simulink model "12_FOC_jieou_fanzhuan_2019b"  (R2019b)
settings: Solver=ode45  StartTime=0.0  StopTime=1  MaxStep=1e-4  RelTol=1e-3  EnableMultiTasking=on
libraries: powerlib x9, simulink x4
settings Model: Creator=uu  LastModifiedBy=李瑾年
settings DataIOCC: LimitDataPoints=on  ReturnWorkspaceOutputs=off
settings OptimizationCC: LifeSpan=inf
settings DebuggingCC: AllowSymbolicDim=off  SFUnexpectedBacktrackingDiag=warning  SFNoUnconditionalDefaultTransitionDiag=warning  ArithmeticOperatorsInVariantConditions=warning
settings ModelReferenceCC: PropagateSignalLabelsOutOfModel=off
settings SFSimCC: SimUseLocalCustomCode=off  CustomCodeUndefinedFunction=UseInterfaceOnly
settings RTWCC: RTWUseLocalCustomCode=off
settings CodeAppCC: StateflowObjectComments=on
settings GRTTargetCC: TargetLangStandard=C89/C90 (ANSI)
settings ConfigComp: CovMetricSettings=dw  CovHtmlReporting=on  CovSaveCumulativeToWorkspaceVar=on  CovSaveSingleToWorkspaceVar=on  CovExternalEMLEnable=off
settings SimscapeCC: SimscapeNormalizeSystem=off

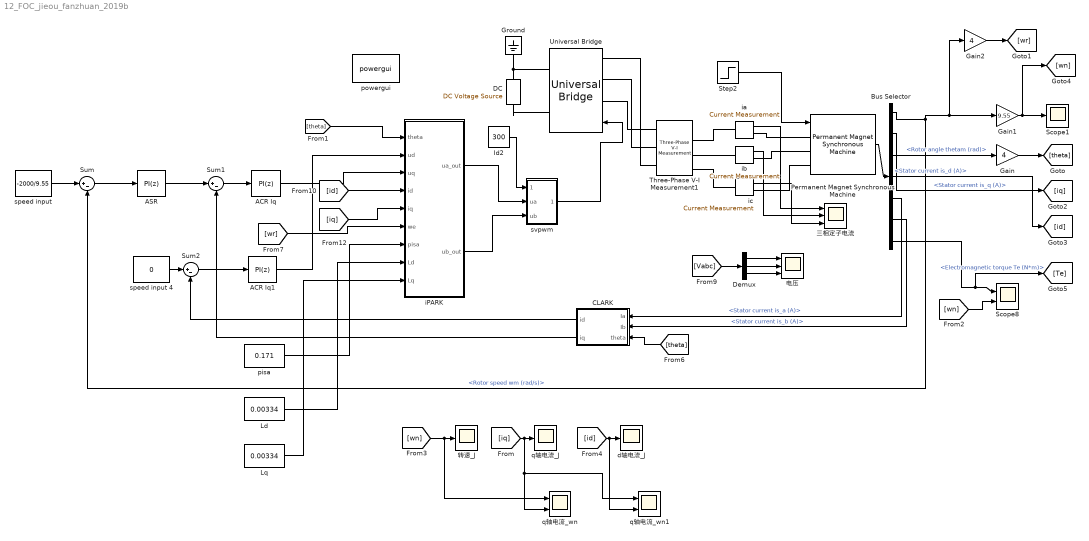
== system 12_FOC_jieou_fanzhuan_2019b ==
  ACR Iq : simulink/Continuous/PID Controller  Controller=PI  Form=Parallel  TimeDomain=Discrete-time  SampleTime=0.0002  IntegratorMethod=Forward Euler  FilterMethod=Forward Euler  ControllerParametersSource=internal  P=15  I=2000  D=0  UseFilter=on  N=100  TunerSelectOption=Transfer Function Based (PID Tuner App)  InitialConditionSource=internal  InitialConditionForIntegrator=0  InitialConditionForFilter=0  DifferentiatorICPrevScaledInput=0  ExternalReset=none  TrackingMode=off  Kt=1  LimitOutput=on  UpperSaturationLimit=320  LowerSaturationLimit=-320  LinearizeAsGain=on  AntiWindupMode=none  Kb=1  POutMin=[]  POutMax=[]  IOutMin=[]  IOutMax=[]  DOutMin=[]  DOutMax=[]  NOutMin=[]  NOutMax=[]  SumOutMin=[]  SumOutMax=[]  SaturationOutMin=[]  SaturationOutMax=[]  PParamMin=[]  PParamMax=[]  IParamMin=[]  IParamMax=[]  DParamMin=[]  DParamMax=[]  NParamMin=[]  NParamMax=[]  KbParamMin=[]  KbParamMax=[]  KtParamMin=[]  KtParamMax=[]  KbOutMin=[]  KbOutMax=[]  KtOutMin=[]  KtOutMax=[]  IntegratorOutMin=[]  IntegratorOutMax=[]  FilterOutMin=[]  FilterOutMax=[]  SumI1OutMin=[]  SumI1OutMax=[]  SumI2OutMin=[]  SumI2OutMax=[]  SumI3OutMin=[]  SumI3OutMax=[]  SumI4OutMin=[]  SumI4OutMax=[]  SumDOutMin=[]  SumDOutMax=[]  DifferentiatorOutMin=[]  DifferentiatorOutMax=[]  FilterDiffOutCoefMin=[]  FilterDiffOutCoefMax=[]  ReciprocalOutMin=[]  ReciprocalOutMax=[]  SumDenOutMin=[]  SumDenOutMax=[]  SumNumOutMin=[]  SumNumOutMax=[]  DivideOutMin=[]  DivideOutMax=[]  IntegratorContinuousStateAttributes=''  IntegratorStateMustResolveToSignalObject=off  IntegratorRTWStateStorageClass=Auto  FilterContinuousStateAttributes=''  FilterStateMustResolveToSignalObject=off  FilterRTWStateStorageClass=Auto  ParallelPVariant=InternalParameters  IdealPVariant=Disabled  IVariant=InternalParameters  DVariant=Disabled  IntegratorVariant=Discrete  SatVariant=Enabled  AWVariant=Passthrough  PCopyVariant=Disabled  TRVariant=Disabled  FdbkBlocksVariant=Forward  IdealPFdbkVariant=Disabled  SatFdbkVariant=Disabled  DerivativeFilterVariant=Disabled  NVariant=Disabled  NCopyVariant=Disabled_SignalSpec  FilterICVariant=Disabled  IntegratorICVariant=InternalICs  ExternalResetVariant=Disabled  TRSumVariant=Passthrough  SumFdbkVariant=Disabled  SumVariant=Sum_PI
  ACR Iq1 : simulink/Continuous/PID Controller  Controller=PI  Form=Parallel  TimeDomain=Discrete-time  SampleTime=0.0002  IntegratorMethod=Forward Euler  FilterMethod=Forward Euler  ControllerParametersSource=internal  P=15  I=2000  D=0  UseFilter=on  N=100  TunerSelectOption=Transfer Function Based (PID Tuner App)  InitialConditionSource=internal  InitialConditionForIntegrator=0  InitialConditionForFilter=0  DifferentiatorICPrevScaledInput=0  ExternalReset=none  TrackingMode=off  Kt=1  LimitOutput=on  UpperSaturationLimit=320  LowerSaturationLimit=-320  LinearizeAsGain=on  AntiWindupMode=none  Kb=1  POutMin=[]  POutMax=[]  IOutMin=[]  IOutMax=[]  DOutMin=[]  DOutMax=[]  NOutMin=[]  NOutMax=[]  SumOutMin=[]  SumOutMax=[]  SaturationOutMin=[]  SaturationOutMax=[]  PParamMin=[]  PParamMax=[]  IParamMin=[]  IParamMax=[]  DParamMin=[]  DParamMax=[]  NParamMin=[]  NParamMax=[]  KbParamMin=[]  KbParamMax=[]  KtParamMin=[]  KtParamMax=[]  KbOutMin=[]  KbOutMax=[]  KtOutMin=[]  KtOutMax=[]  IntegratorOutMin=[]  IntegratorOutMax=[]  FilterOutMin=[]  FilterOutMax=[]  SumI1OutMin=[]  SumI1OutMax=[]  SumI2OutMin=[]  SumI2OutMax=[]  SumI3OutMin=[]  SumI3OutMax=[]  SumI4OutMin=[]  SumI4OutMax=[]  SumDOutMin=[]  SumDOutMax=[]  DifferentiatorOutMin=[]  DifferentiatorOutMax=[]  FilterDiffOutCoefMin=[]  FilterDiffOutCoefMax=[]  ReciprocalOutMin=[]  ReciprocalOutMax=[]  SumDenOutMin=[]  SumDenOutMax=[]  SumNumOutMin=[]  SumNumOutMax=[]  DivideOutMin=[]  DivideOutMax=[]  IntegratorContinuousStateAttributes=''  IntegratorStateMustResolveToSignalObject=off  IntegratorRTWStateStorageClass=Auto  FilterContinuousStateAttributes=''  FilterStateMustResolveToSignalObject=off  FilterRTWStateStorageClass=Auto  ParallelPVariant=InternalParameters  IdealPVariant=Disabled  IVariant=InternalParameters  DVariant=Disabled  IntegratorVariant=Discrete  SatVariant=Enabled  AWVariant=Passthrough  PCopyVariant=Disabled  TRVariant=Disabled  FdbkBlocksVariant=Forward  IdealPFdbkVariant=Disabled  SatFdbkVariant=Disabled  DerivativeFilterVariant=Disabled  NVariant=Disabled  NCopyVariant=Disabled_SignalSpec  FilterICVariant=Disabled  IntegratorICVariant=InternalICs  ExternalResetVariant=Disabled  TRSumVariant=Passthrough  SumFdbkVariant=Disabled  SumVariant=Sum_PI
  ASR : simulink/Continuous/PID Controller  Controller=PI  Form=Parallel  TimeDomain=Discrete-time  SampleTime=0.0002  IntegratorMethod=Forward Euler  FilterMethod=Forward Euler  ControllerParametersSource=internal  P=6  I=3  D=0  UseFilter=on  N=100  TunerSelectOption=Transfer Function Based (PID Tuner App)  InitialConditionSource=internal  InitialConditionForIntegrator=0  InitialConditionForFilter=0  DifferentiatorICPrevScaledInput=0  ExternalReset=none  TrackingMode=off  Kt=1  LimitOutput=on  UpperSaturationLimit=25  LowerSaturationLimit=-25  LinearizeAsGain=on  AntiWindupMode=none  Kb=1  POutMin=[]  POutMax=[]  IOutMin=[]  IOutMax=[]  DOutMin=[]  DOutMax=[]  NOutMin=[]  NOutMax=[]  SumOutMin=[]  SumOutMax=[]  SaturationOutMin=[]  SaturationOutMax=[]  PParamMin=[]  PParamMax=[]  IParamMin=[]  IParamMax=[]  DParamMin=[]  DParamMax=[]  NParamMin=[]  NParamMax=[]  KbParamMin=[]  KbParamMax=[]  KtParamMin=[]  KtParamMax=[]  KbOutMin=[]  KbOutMax=[]  KtOutMin=[]  KtOutMax=[]  IntegratorOutMin=[]  IntegratorOutMax=[]  FilterOutMin=[]  FilterOutMax=[]  SumI1OutMin=[]  SumI1OutMax=[]  SumI2OutMin=[]  SumI2OutMax=[]  SumI3OutMin=[]  SumI3OutMax=[]  SumI4OutMin=[]  SumI4OutMax=[]  SumDOutMin=[]  SumDOutMax=[]  DifferentiatorOutMin=[]  DifferentiatorOutMax=[]  FilterDiffOutCoefMin=[]  FilterDiffOutCoefMax=[]  ReciprocalOutMin=[]  ReciprocalOutMax=[]  SumDenOutMin=[]  SumDenOutMax=[]  SumNumOutMin=[]  SumNumOutMax=[]  DivideOutMin=[]  DivideOutMax=[]  IntegratorContinuousStateAttributes=''  IntegratorStateMustResolveToSignalObject=off  IntegratorRTWStateStorageClass=Auto  FilterContinuousStateAttributes=''  FilterStateMustResolveToSignalObject=off  FilterRTWStateStorageClass=Auto  ParallelPVariant=InternalParameters  IdealPVariant=Disabled  IVariant=InternalParameters  DVariant=Disabled  IntegratorVariant=Discrete  SatVariant=Enabled  AWVariant=Passthrough  PCopyVariant=Disabled  TRVariant=Disabled  FdbkBlocksVariant=Forward  IdealPFdbkVariant=Disabled  SatFdbkVariant=Disabled  DerivativeFilterVariant=Disabled  NVariant=Disabled  NCopyVariant=Disabled_SignalSpec  FilterICVariant=Disabled  IntegratorICVariant=InternalICs  ExternalResetVariant=Disabled  TRSumVariant=Passthrough  SumFdbkVariant=Disabled  SumVariant=Sum_PI
  Bus Selector : BusSelector  OutputSignals=Rotor speed wm (rad/s),Rotor angle thetam (rad),Stator current is_q (A),Stator current is_d (A),Stator current is_a (A),Stator current is_b (A),Electromagnetic torque Te (N*m)
  CLARK : MATLAB Function  TreatAsAtomicUnit=on
  "DC " : powerlib/Electrical Sources/DC Voltage Source  Amplitude=300  Measurements=None
      settings: SourceProductName=Simscape Electrical
  Demux : Demux  Outputs=3
  Gain : Gain  Gain=4
  Gain1 : Gain  Gain=9.55
  Gain2 : Gain  Gain=4
  Ground : powerlib/Elements/Ground  LConnTagsString=a
      settings: SourceProductName=Simscape Electrical
  Id2 : Constant  Value=300
  Ld : Constant  Value=0.00334
  Lq : Constant  Value=0.00334
  Permanent Magnet Synchronous Machine : powerlib/Machines/Permanent Magnet Synchronous Machine  NbPhases=3  FluxDistribution=Sinusoidal  RotorType=Round  MechanicalLoad=Torque Tm  PresetModel="06:  10 Nm 300 Vdc 2300 RPM - 14.2 Nm"  ShowDetailedParameters=on  MeasurementBus=off  Resistance=0.4578  Inductance=8.5e-3  dqInductances=[2.1e-3,2.1e-3]  La=0.00334  MachineConstant=Flux linkage established by magnets (V.s)  Flux=0.171  VoltageCst=124.0639  TorqueCst=1.026  Flat=120  Mechanical=[0.001469 0.0003035 4 0]  PolePairs=4  InitialConditions=[0,0, 0,0]  InitialConditions5ph=[0 0 0 0 0 0]  RefAngle=Aligned with phase A axis (original Park)  IterativeDiscreteModel=Trapezoidal non iterative  TsBlock=-1  TsPowergui=0
  Scope1 : Scope
  Scope8 : Scope  NumInputPorts=2
  Step2 : Step  Time=0.25  After=13  SampleTime=0
  Sum : Sum  Inputs=|+-
  Sum1 : Sum  Inputs=|+-
  Sum2 : Sum  Inputs=|+-
  Three-Phase V-I Measurement1 : powerlib/Measurements/Three-Phase V-I Measurement  VoltageMeasurement=phase-to-ground  SetLabelV=on  LabelV=Vabc  Vpu=off  VpuLL=off  CurrentMeasurement=yes  SetLabelI=off  LabelI=Iabc  Ipu=off  Pbase=100e6  Vbase=500e3  OutputType=Complex  PhasorSimulation=off  PSBequivalent=0
      settings: SourceProductName=Simscape Electrical
  Universal Bridge : powerlib/Power Electronics/Universal Bridge  Arms=3  SnubberResistance=1e5  SnubberCapacitance=inf  Device=IGBT / Diodes  Ron=1e-3  Lon=0  ForwardVoltages="[  0  0  ]"  ForwardVoltage=0  GTOparameters=[ 10e-6 , 20e-6 ]  IGBTparameters=[ 1e-6 , 2e-6 ]  Measurements=None  Measurements_2=None  converterType=Rectifier
      settings: SourceProductName=Simscape Electrical
  "d轴电流_J " : Scope
  iPARK : MATLAB Function  TreatAsAtomicUnit=on
  ia : powerlib/Measurements/Current Measurement  PhasorSimulation=off  OutputType=Complex  PSBequivalent=0
      settings: SourceProductName=Simscape Electrical
  ib : powerlib/Measurements/Current Measurement  PhasorSimulation=off  OutputType=Complex  PSBequivalent=0
      settings: SourceProductName=Simscape Electrical
  ic : powerlib/Measurements/Current Measurement  PhasorSimulation=off  OutputType=Complex  PSBequivalent=0
      settings: SourceProductName=Simscape Electrical
  pisa : Constant  Value=0.171
  powergui : powerlib/powergui  Priority=1  SimulationMode=Discrete  SampleTime=1e-6  frequency=60  Iterations=50  frequencyindice=0  Pbase=100e6  ErrMax=1e-4  UnitsV=kV  UnitsW=MW  buscounter=0  FunctionMessages=off  echomessages=off  EnableUseOfTLC=off  CurrentSourceSwitches=off  DisableSnubberDevices=off  DisableRonSwitches=off  DisableVfSwitches=off  DisplayEquations=off  AutomaticDiscreteSolvers=off  SolverType=Tustin/Backward Euler (TBE)  Interpol=off  ExternalGateDelay=off  methode=off  Ts=100  x0status=blocks  SPID=off  SwTol=0  HookPort=off  NonlinearTolerance=1e-4  nMaxIteration=100  ContinueOnMaxIteration=off  RestoreLinks=warning  ResistiveCurrentMeasurement=off  Frange=[0:2:500]  Ylog=off  Xlog=on  ShowGrid=off  save=off  variable=ZData  structure=ScopeData  ZoomFFT=off  StartTime=0.0  cycles=1  DisplayStyle=1  fundamental=60  FreqAxis=off  MaxFrequency=1000  frequencyindicesteady=1  RmsSteady=1  display=off
      settings: SourceProductName=Simscape Electrical
  q轴电流_J : Scope
  q轴电流_wn : Scope  NumInputPorts=2
  q轴电流_wn1 : Scope  NumInputPorts=2
  "speed input " : Constant  Value=-2000/9.55
  speed input 4 : Constant  Value=0
  "svpwm " : Subsystem
  三相定子电流 : Scope  NumInputPorts=3
  电压 : Scope  NumInputPorts=3
  转速_J : Scope
  wires:
  Bus Selector/1 -> Gain2/1, Gain1/1, Sum/2  "<Rotor speed wm (rad/s)>"
  Bus Selector/2 -> Gain/1  "<Rotor angle thetam (rad)>"
  Sum2/1 -> ACR Iq1/1
  Sum1/1 -> ACR Iq/1
  Gain/1 -> [theta]
  "speed input "/1 -> Sum/1
  Gain1/1 -> [wn], Scope1/1
  Bus Selector/3 -> [iq]  "<Stator current is_q (A)>"
  Bus Selector/4 -> [id]  "<Stator current is_d (A)>"
  Bus Selector/5 -> CLARK/1(Ia)  "<Stator current is_a (A)>"
  Bus Selector/6 -> CLARK/2(Ib)  "<Stator current is_b (A)>"
  ib/1 -> 三相定子电流/2
  Bus Selector/7 -> [Te], Scope8/1  "<Electromagnetic torque Te (N*m)>"
  CLARK/1(id) -> Sum2/2
  [theta] -> iPARK/1(theta)
  CLARK/2(iq) -> Sum1/2
  [wn] -> Scope8/2
  ia/1 -> 三相定子电流/1
  ic/1 -> 三相定子电流/3
  Id2/1 -> "svpwm "/1(Udc)
  iPARK/1(ua_out) -> "svpwm "/2(ua)
  iPARK/2(ub_out) -> "svpwm "/3(ub)
  "svpwm "/1(Out1) -> Universal Bridge/1
  [wn] -> q轴电流_wn/1, 转速_J/1
  [iq] -> q轴电流_wn1/1, q轴电流_wn/2, q轴电流_J/1
  [id] -> q轴电流_wn1/2, "d轴电流_J "/1
  [wr] -> iPARK/6(we)
  pisa/1 -> iPARK/7(pisa)
  Ld/1 -> iPARK/8(Ld)
  Lq/1 -> iPARK/9(Lq)
  speed input 4/1 -> Sum2/1
  Permanent Magnet Synchronous Machine/1 -> Bus Selector/1
  Sum/1 -> ASR/1
  ASR/1 -> Sum1/1
  [Vabc] -> Demux/1
  Demux/1 -> 电压/1
  Demux/3 -> 电压/3
  Demux/2 -> 电压/2
  ACR Iq/1 -> iPARK/3(uq)
  ACR Iq1/1 -> iPARK/2(ud)
  [id] -> iPARK/4(id)
  [iq] -> iPARK/5(iq)
  [theta] -> CLARK/3(theta)
  Gain2/1 -> [wr]
  Step2/1 -> Permanent Magnet Synchronous Machine/1
  connections:
  "DC "/RConn1 -- Universal Bridge/RConn1
  "DC "/LConn1 -- Ground/LConn1 -- Universal Bridge/RConn2
  Permanent Magnet Synchronous Machine/LConn1 -- ia/RConn1
  Permanent Magnet Synchronous Machine/LConn2 -- ib/RConn1
  Permanent Magnet Synchronous Machine/LConn3 -- ic/RConn1
  Universal Bridge/LConn3 -- Three-Phase V-I Measurement1/LConn3
  Universal Bridge/LConn2 -- Three-Phase V-I Measurement1/LConn2
  Universal Bridge/LConn1 -- Three-Phase V-I Measurement1/LConn1
  Three-Phase V-I Measurement1/RConn1 -- ia/LConn1
  Three-Phase V-I Measurement1/RConn2 -- ib/LConn1
  Three-Phase V-I Measurement1/RConn3 -- ic/LConn1

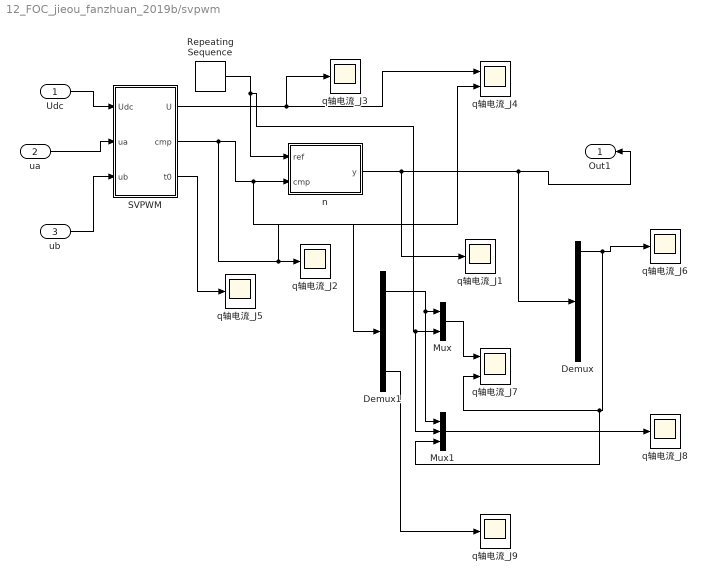
== system 12_FOC_jieou_fanzhuan_2019b/svpwm  ==
  Udc : Inport
  ua : Inport  Port=2
  ub : Inport  Port=3
  Demux : Demux  Outputs=6
  Demux1 : Demux  Outputs=3
  Mux : Mux  Inputs=2
  Mux1 : Mux  Inputs=3
  Repeating Sequence : simulink/Sources/Repeating Sequence  rep_seq_t=[0 0.0001 0.0002]  rep_seq_y=[0 1 0]
  SVPWM : MATLAB Function  TreatAsAtomicUnit=on
  n : MATLAB Function  TreatAsAtomicUnit=on
  q轴电流_J{1..3,5..6,8..9} (7 alike) : Scope
  q轴电流_J4 : Scope  NumInputPorts=2
  q轴电流_J7 : Scope  NumInputPorts=2
  Out1 : Outport
  wires:
  Repeating Sequence/1 -> Mux1/2, Mux/2, n/1(ref)
  SVPWM/2(cmp) -> q轴电流_J4/2, q轴电流_J2/1, Demux1/1, n/2(cmp)
  Udc/1 -> SVPWM/1(Udc)
  n/1(y) -> q轴电流_J1/1, Demux/1, Out1/1
  ua/1 -> SVPWM/2(ua)
  ub/1 -> SVPWM/3(ub)
  SVPWM/1(U) -> q轴电流_J4/1, q轴电流_J3/1
  SVPWM/3(t0) -> q轴电流_J5/1
  Demux/1 -> Mux1/3, q轴电流_J7/2, q轴电流_J6/1
  Demux1/1 -> Mux1/1, Mux/1
  Mux/1 -> q轴电流_J7/1
  Mux1/1 -> q轴电流_J8/1
  Demux1/3 -> q轴电流_J9/1

== matlab function 12_FOC_jieou_fanzhuan_2019b/iPARK ==
  data: ua_out output; theta input; ud input; uq input; ub_out output; id input; iq input; we input; pisa input; Ld input; Lq input
function [ua_out,ub_out]   = fcn(theta,ud,uq,id,iq,we,pisa,Ld,Lq)



ud=ud-iq*we*Lq;
uq=uq+id*we*Ld+we*pisa;
uaa=ud;
ubb=uq;
theta1=sin(theta);
 
ua_out=ud*cos(theta)-uq*sin(theta);
ub_out=ud*sin(theta)+uq*cos(theta);
  

end

== matlab function 12_FOC_jieou_fanzhuan_2019b/CLARK ==
  data: Ia input; id output; iq output; Ib input; theta input
function [id,iq] = fcn(Ia,Ib,theta)
%#codegen

 ia=sqrt(2/3)*sqrt(3/2)*Ia;               % 3/2变换  N3/N2 = 2/3   且  ia + ib + ic = 0 
 ib=sqrt(2/3)*(1/sqrt(2)*Ia+sqrt(2)*Ib);
 id=ia*cos(theta)+ib*sin(theta);          % 2/2变换
 iq=-ia*sin(theta)+ib*cos(theta);
end

== matlab function 12_FOC_jieou_fanzhuan_2019b/svpwm /SVPWM ==
  data: U output; Udc input; ua input; cmp output; ub input; t0 output
function [U,cmp,t0]= SVPWM(Udc,ua,ub)
%#codegen
Ta=0.5;
Tb=0.5;
Tc=0.5;
%判断所在扇区
U=ua+1j*ub;                                        %将得到的两相静止坐标系的ua 和 ub 变为虚数形式  用angle计算出角度
duty=min(1,abs(U)*sqrt(3)/Udc);   %防止过调制               防止超过SVPWM的正六边形  最大相电压幅值  sqrt(3)/3*udc
                                                           %abs() 求复数幅值  
theta=mod(angle(U),2*pi);  %角度除以2π取余
sector=floor(theta/(pi/3));                                %角度除以π/3向下取整 判断所在扇区  例如1/3pi在 I扇区
theta=theta-sector*pi/3;                                   %floor()  取整   比如 
%计算基本矢量作用时间                                       
t1=duty*sin(pi/3-theta);                                   % 两个电压矢量作用时间                           
t2=duty*sin(theta);
%设置sector1,3,5扇区的    交换t1，t2值  
if (sector==1)||(sector==3)||(sector==5)
    ttemp=t1;
    t1=t2;
    t2=ttemp;
end
%计算中间变量
taon=(1-t1-t2)/4;                         % 除去基本矢量所去的时间  再乘 1/4
tbon=taon+t1/2;                           % 基本矢量1作用时间 乘 1/2  + 上
tcon=tbon+t2/2;                           % 基本矢量2作用时间 乘 1/2  + 上
t0=taon;
%切换时间
switch sector                             
    case 0                              % 如果在 I 区 
        Ta=taon;
        Tb=tbon;
        Tc=tcon;
    case 1
        Ta=tbon;
        Tb=taon;
        Tc=tcon;
    case 2
        Ta=tcon;
        Tb=taon;
        Tc=tbon;
    case 3
        Ta=tcon;
        Tb=tbon;
        Tc=taon;
    case 4
        Ta=tbon;
        Tb=tcon;
        Tc=taon;
    case 5
        Ta=taon;
        Tb=tcon;
        Tc=tbon;
end
t=[Ta,Tb,Tc];
cmp=2*t;
end

== matlab function 12_FOC_jieou_fanzhuan_2019b/svpwm /n ==
  data: ref input; y output; cmp input
function y  = fcn(ref,cmp)
%#codegen
Ta1=0;
Ta2=0;
Tb1=0;
Tb2=0;
Tc1=0;
Tc2=0;
if ref>=cmp(1)            % ref 就是一个三角波发生器  A相PWM波形成  累加的过程中 Taon 大于了三角波  就 A相下桥臂通 上桥臂关
    Ta1=1;
    Ta2=0;
elseif ref<cmp(1)
    Ta1=0;
    Ta2=1;
end

if ref>=cmp(2)
    Tb1=1;
    Tb2=0;
elseif ref<cmp(2)
    Tb1=0;
    Tb2=1;
end

if ref>=cmp(3)
    Tc1=1;
    Tc2=0;
elseif ref<cmp(3)
    Tc1=0;
    Tc2=1;
end

y=[Ta1;Ta2;Tb1;Tb2;Tc1;Tc2];
